simulink model "ng_pv_dynamic_dbus_p_1_sm_ng"  (Simulink 8.8)
settings: Solver=ode4  StartTime=0.0  StopTime=inf  FixedStep=0.000125  RelTol=1e-3  EnableMultiTasking=on
PreLoadFcn:
  | Ts=125e-6;Core_Num = 0; np=1; nq=1; Vmin=.9;
PostLoadFcn:
  | Ts=125e-6;Core_Num = 0; np=1; nq=1; Vmin=.9;
InitFcn:
  | Ts=125e-6;Core_Num = 0; np=1; nq=1; Vmin=.9;
undefined symbols (not defined in the file or in its folder): another_event_name, DiscIntNeverNeededParam, I, j, Left, my_event_name, Right, type, V, X
libraries: powerlib x316, simulink_extras x78, powerlib_meascontrol x47, ssn_lib x9, opal_lib x5, powerlib_extras x3, simulink x3, artemis x1, rtio_opalrt_ml605ex1 x1, rtlab x1, rtio_spectracom x1
(part 3 of 11)

== system ng_pv_dynamic_dbus_p_1_sm_ng/SM_NG/Dynamic Load BCDC1 ==
  P : Inport
  Q : Inport  Port=2
  Ground27 : powerlib/Elements/Ground  LConnTagsString=a
  Single-Phase Dynamic Load1 : Subsystem  DialogController=POWERSYS.PowerSysDialog  mask(Single-Phase Dynamic Load){NominalVoltage=|, ActiveReactivePowers=[664828.3847 359143.0862], PositiveSequence=[1 0], ExternalControl=on, NpNq=[np nq], TimeConstants=[0  0  0  0], MinimumVoltage=Vmin, LoadFlowParameters=[4,0,0,0,0]}
      mask NominalVoltage=|
      | [7967.4337
      | 60]
      mask prompts: NominalVoltage "Nominal voltage and frequency  [Vn(Vrms) fn(Hz)]:"; ActiveReactivePowers "Active and reactive power at initial voltage [Po(W) Qo(var)]:"; PositiveSequence "Initial voltage Vo [Mag(pu) Phase (deg.)]:"; ExternalControl "External control of PQ"; NpNq "Parameters [ np  nq ]:"; TimeConstants "Time constants [Tp1 Tp2 Tq1 Tq2]  (s):"; MinimumVoltage "Minimum voltage Vmin (pu):"; LoadFlowParameters "Load Flow parameters"
      mask help:
      | Implements a single-phase dynamic load. Active  power P and reactive
      | power Q absorbed by the load vary as function of voltage V  according to the
      | following equations:
      |
      |   If V>Vmin, P and Q vary as follows:
      |        P = Po * (V/Vo)^np * (1+Tp1.s)/(1+Tp2.s)
      |        Q = Qo * (V/Vo)^nq * (1+Tq1.s)/(1+Tq2.s)
      |   if V<Vmin
      |      Same equations with np=nq=2 (constant impedance load)
      mask init: same as ng_pv_dynamic_dbus_p_1_sm_ng/SM_NG/Single-Phase Dynamic Load32
      mask Help: helpview(psbhelp)
      mask Callback ExternalControl: powericon('ThreePhaseDynamicLoadCback',gcb);
      mask Display:
      | plot(-45,-45,45,45,[0,9,18,24,29,30,29,24,18,9,0,-9,-18,-24,-29,-30,-29,-24,-18,-9,0]*.9,[30,29,24,18,9,0,-9,-18,-24,-29,-30,-29,-24,-18,-9,0,9,18,24,29,30]*.9)
      | plot([0,0,10,0,-10,0]*1.1,[15,-5,-5,-15,-5,-5]*1.1)
  Single-Phase Dynamic Load2 : Subsystem  DialogController=POWERSYS.PowerSysDialog  mask(Single-Phase Dynamic Load){NominalVoltage=|, ActiveReactivePowers=[192621.3908 153291.9797], PositiveSequence=[1 0], ExternalControl=on, NpNq=[np nq], TimeConstants=[0  0  0  0], MinimumVoltage=Vmin, LoadFlowParameters=[4,0,0,0,0]}
      mask NominalVoltage=|
      | [7967.4337
      | 60]
      mask prompts: NominalVoltage "Nominal voltage and frequency  [Vn(Vrms) fn(Hz)]:"; ActiveReactivePowers "Active and reactive power at initial voltage [Po(W) Qo(var)]:"; PositiveSequence "Initial voltage Vo [Mag(pu) Phase (deg.)]:"; ExternalControl "External control of PQ"; NpNq "Parameters [ np  nq ]:"; TimeConstants "Time constants [Tp1 Tp2 Tq1 Tq2]  (s):"; MinimumVoltage "Minimum voltage Vmin (pu):"; LoadFlowParameters "Load Flow parameters"
      mask help:
      | Implements a single-phase dynamic load. Active  power P and reactive
      | power Q absorbed by the load vary as function of voltage V  according to the
      | following equations:
      |
      |   If V>Vmin, P and Q vary as follows:
      |        P = Po * (V/Vo)^np * (1+Tp1.s)/(1+Tp2.s)
      |        Q = Qo * (V/Vo)^nq * (1+Tq1.s)/(1+Tq2.s)
      |   if V<Vmin
      |      Same equations with np=nq=2 (constant impedance load)
      mask init: same as ng_pv_dynamic_dbus_p_1_sm_ng/SM_NG/Single-Phase Dynamic Load32
      mask Help: helpview(psbhelp)
      mask Callback ExternalControl: powericon('ThreePhaseDynamicLoadCback',gcb);
      mask Display:
      | plot(-45,-45,45,45,[0,9,18,24,29,30,29,24,18,9,0,-9,-18,-24,-29,-30,-29,-24,-18,-9,0]*.9,[30,29,24,18,9,0,-9,-18,-24,-29,-30,-29,-24,-18,-9,0,9,18,24,29,30]*.9)
      | plot([0,0,10,0,-10,0]*1.1,[15,-5,-5,-15,-5,-5]*1.1)
  Single-Phase Dynamic Load9 : Subsystem  DialogController=POWERSYS.PowerSysDialog  mask(Single-Phase Dynamic Load){NominalVoltage=|, ActiveReactivePowers=[324233.2017 230913.2561], PositiveSequence=[1 0], ExternalControl=on, NpNq=[np nq], TimeConstants=[0  0  0  0], MinimumVoltage=Vmin, LoadFlowParameters=[4,0,0,0,0]}
      mask NominalVoltage=|
      | [7967.4337
      | 60]
      mask prompts: NominalVoltage "Nominal voltage and frequency  [Vn(Vrms) fn(Hz)]:"; ActiveReactivePowers "Active and reactive power at initial voltage [Po(W) Qo(var)]:"; PositiveSequence "Initial voltage Vo [Mag(pu) Phase (deg.)]:"; ExternalControl "External control of PQ"; NpNq "Parameters [ np  nq ]:"; TimeConstants "Time constants [Tp1 Tp2 Tq1 Tq2]  (s):"; MinimumVoltage "Minimum voltage Vmin (pu):"; LoadFlowParameters "Load Flow parameters"
      mask help:
      | Implements a single-phase dynamic load. Active  power P and reactive
      | power Q absorbed by the load vary as function of voltage V  according to the
      | following equations:
      |
      |   If V>Vmin, P and Q vary as follows:
      |        P = Po * (V/Vo)^np * (1+Tp1.s)/(1+Tp2.s)
      |        Q = Qo * (V/Vo)^nq * (1+Tq1.s)/(1+Tq2.s)
      |   if V<Vmin
      |      Same equations with np=nq=2 (constant impedance load)
      mask init: same as ng_pv_dynamic_dbus_p_1_sm_ng/SM_NG/Single-Phase Dynamic Load32
      mask Help: helpview(psbhelp)
      mask Callback ExternalControl: powericon('ThreePhaseDynamicLoadCback',gcb);
      mask Display:
      | plot(-45,-45,45,45,[0,9,18,24,29,30,29,24,18,9,0,-9,-18,-24,-29,-30,-29,-24,-18,-9,0]*.9,[30,29,24,18,9,0,-9,-18,-24,-29,-30,-29,-24,-18,-9,0,9,18,24,29,30]*.9)
      | plot([0,0,10,0,-10,0]*1.1,[15,-5,-5,-15,-5,-5]*1.1)
  A : PMIOPort  Port=1  Side=Right
  B : PMIOPort  Port=2  Side=Right
  C : PMIOPort  Port=3  Side=Right
  wires:
  P/1 -> Single-Phase Dynamic Load2/1(P), Single-Phase Dynamic Load1/1(P), Single-Phase Dynamic Load9/1(P)
  Q/1 -> Single-Phase Dynamic Load1/2(Q), Single-Phase Dynamic Load2/2(Q), Single-Phase Dynamic Load9/2(Q)
  connections:
  Single-Phase Dynamic Load9/LConn2 -- Single-Phase Dynamic Load1/LConn2 -- Ground27/LConn1 -- Single-Phase Dynamic Load2/LConn2
  A/RConn1 -- Single-Phase Dynamic Load9/LConn1
  Single-Phase Dynamic Load2/LConn1 -- C/RConn1
  Single-Phase Dynamic Load1/LConn1 -- B/RConn1

== system ng_pv_dynamic_dbus_p_1_sm_ng/SM_NG/Dynamic Load BCDC2 ==
  P : Inport
  Q : Inport  Port=2
  Ground27 : powerlib/Elements/Ground  LConnTagsString=a
  Single-Phase Dynamic Load1 : Subsystem  DialogController=POWERSYS.PowerSysDialog  mask(Single-Phase Dynamic Load){NominalVoltage=|, ActiveReactivePowers=[934247.1199 467237.5312], PositiveSequence=[1 0], ExternalControl=on, NpNq=[np nq], TimeConstants=[0  0  0  0], MinimumVoltage=Vmin, LoadFlowParameters=[4,0,0,0,0]}
      mask NominalVoltage=|
      | [7967.4337
      | 60]
      mask prompts: NominalVoltage "Nominal voltage and frequency  [Vn(Vrms) fn(Hz)]:"; ActiveReactivePowers "Active and reactive power at initial voltage [Po(W) Qo(var)]:"; PositiveSequence "Initial voltage Vo [Mag(pu) Phase (deg.)]:"; ExternalControl "External control of PQ"; NpNq "Parameters [ np  nq ]:"; TimeConstants "Time constants [Tp1 Tp2 Tq1 Tq2]  (s):"; MinimumVoltage "Minimum voltage Vmin (pu):"; LoadFlowParameters "Load Flow parameters"
      mask help:
      | Implements a single-phase dynamic load. Active  power P and reactive
      | power Q absorbed by the load vary as function of voltage V  according to the
      | following equations:
      |
      |   If V>Vmin, P and Q vary as follows:
      |        P = Po * (V/Vo)^np * (1+Tp1.s)/(1+Tp2.s)
      |        Q = Qo * (V/Vo)^nq * (1+Tq1.s)/(1+Tq2.s)
      |   if V<Vmin
      |      Same equations with np=nq=2 (constant impedance load)
      mask init: same as ng_pv_dynamic_dbus_p_1_sm_ng/SM_NG/Single-Phase Dynamic Load32
      mask Help: helpview(psbhelp)
      mask Callback ExternalControl: powericon('ThreePhaseDynamicLoadCback',gcb);
      mask Display:
      | plot(-45,-45,45,45,[0,9,18,24,29,30,29,24,18,9,0,-9,-18,-24,-29,-30,-29,-24,-18,-9,0]*.9,[30,29,24,18,9,0,-9,-18,-24,-29,-30,-29,-24,-18,-9,0,9,18,24,29,30]*.9)
      | plot([0,0,10,0,-10,0]*1.1,[15,-5,-5,-15,-5,-5]*1.1)
  Single-Phase Dynamic Load2 : Subsystem  DialogController=POWERSYS.PowerSysDialog  mask(Single-Phase Dynamic Load){NominalVoltage=|, ActiveReactivePowers=[586764.5672 402164.5376], PositiveSequence=[1 0], ExternalControl=on, NpNq=[np nq], TimeConstants=[0  0  0  0], MinimumVoltage=Vmin, LoadFlowParameters=[4,0,0,0,0]}
      mask NominalVoltage=|
      | [7967.4337
      | 60]
      mask prompts: NominalVoltage "Nominal voltage and frequency  [Vn(Vrms) fn(Hz)]:"; ActiveReactivePowers "Active and reactive power at initial voltage [Po(W) Qo(var)]:"; PositiveSequence "Initial voltage Vo [Mag(pu) Phase (deg.)]:"; ExternalControl "External control of PQ"; NpNq "Parameters [ np  nq ]:"; TimeConstants "Time constants [Tp1 Tp2 Tq1 Tq2]  (s):"; MinimumVoltage "Minimum voltage Vmin (pu):"; LoadFlowParameters "Load Flow parameters"
      mask help:
      | Implements a single-phase dynamic load. Active  power P and reactive
      | power Q absorbed by the load vary as function of voltage V  according to the
      | following equations:
      |
      |   If V>Vmin, P and Q vary as follows:
      |        P = Po * (V/Vo)^np * (1+Tp1.s)/(1+Tp2.s)
      |        Q = Qo * (V/Vo)^nq * (1+Tq1.s)/(1+Tq2.s)
      |   if V<Vmin
      |      Same equations with np=nq=2 (constant impedance load)
      mask init: same as ng_pv_dynamic_dbus_p_1_sm_ng/SM_NG/Single-Phase Dynamic Load32
      mask Help: helpview(psbhelp)
      mask Callback ExternalControl: powericon('ThreePhaseDynamicLoadCback',gcb);
      mask Display:
      | plot(-45,-45,45,45,[0,9,18,24,29,30,29,24,18,9,0,-9,-18,-24,-29,-30,-29,-24,-18,-9,0]*.9,[30,29,24,18,9,0,-9,-18,-24,-29,-30,-29,-24,-18,-9,0,9,18,24,29,30]*.9)
      | plot([0,0,10,0,-10,0]*1.1,[15,-5,-5,-15,-5,-5]*1.1)
  Single-Phase Dynamic Load9 : Subsystem  DialogController=POWERSYS.PowerSysDialog  mask(Single-Phase Dynamic Load){NominalVoltage=|, ActiveReactivePowers=[473340.7231 336359.2548], PositiveSequence=[1 0], ExternalControl=on, NpNq=[np nq], TimeConstants=[0  0  0  0], MinimumVoltage=Vmin, LoadFlowParameters=[4,0,0,0,0]}
      mask NominalVoltage=|
      | [7967.4337
      | 60]
      mask prompts: NominalVoltage "Nominal voltage and frequency  [Vn(Vrms) fn(Hz)]:"; ActiveReactivePowers "Active and reactive power at initial voltage [Po(W) Qo(var)]:"; PositiveSequence "Initial voltage Vo [Mag(pu) Phase (deg.)]:"; ExternalControl "External control of PQ"; NpNq "Parameters [ np  nq ]:"; TimeConstants "Time constants [Tp1 Tp2 Tq1 Tq2]  (s):"; MinimumVoltage "Minimum voltage Vmin (pu):"; LoadFlowParameters "Load Flow parameters"
      mask help:
      | Implements a single-phase dynamic load. Active  power P and reactive
      | power Q absorbed by the load vary as function of voltage V  according to the
      | following equations:
      |
      |   If V>Vmin, P and Q vary as follows:
      |        P = Po * (V/Vo)^np * (1+Tp1.s)/(1+Tp2.s)
      |        Q = Qo * (V/Vo)^nq * (1+Tq1.s)/(1+Tq2.s)
      |   if V<Vmin
      |      Same equations with np=nq=2 (constant impedance load)
      mask init: same as ng_pv_dynamic_dbus_p_1_sm_ng/SM_NG/Single-Phase Dynamic Load32
      mask Help: helpview(psbhelp)
      mask Callback ExternalControl: powericon('ThreePhaseDynamicLoadCback',gcb);
      mask Display:
      | plot(-45,-45,45,45,[0,9,18,24,29,30,29,24,18,9,0,-9,-18,-24,-29,-30,-29,-24,-18,-9,0]*.9,[30,29,24,18,9,0,-9,-18,-24,-29,-30,-29,-24,-18,-9,0,9,18,24,29,30]*.9)
      | plot([0,0,10,0,-10,0]*1.1,[15,-5,-5,-15,-5,-5]*1.1)
  A : PMIOPort  Port=1  Side=Right
  B : PMIOPort  Port=2  Side=Right
  C : PMIOPort  Port=3  Side=Right
  wires:
  P/1 -> Single-Phase Dynamic Load2/1(P), Single-Phase Dynamic Load1/1(P), Single-Phase Dynamic Load9/1(P)
  Q/1 -> Single-Phase Dynamic Load1/2(Q), Single-Phase Dynamic Load2/2(Q), Single-Phase Dynamic Load9/2(Q)
  connections:
  Single-Phase Dynamic Load9/LConn2 -- Single-Phase Dynamic Load1/LConn2 -- Ground27/LConn1 -- Single-Phase Dynamic Load2/LConn2
  A/RConn1 -- Single-Phase Dynamic Load9/LConn1
  Single-Phase Dynamic Load2/LConn1 -- C/RConn1
  Single-Phase Dynamic Load1/LConn1 -- B/RConn1

== system ng_pv_dynamic_dbus_p_1_sm_ng/SM_NG/Dynamic Load BCDC3 ==
  P : Inport
  Q : Inport  Port=2
  Ground27 : powerlib/Elements/Ground  LConnTagsString=a
  Single-Phase Dynamic Load1 : Subsystem  DialogController=POWERSYS.PowerSysDialog  mask(Single-Phase Dynamic Load){NominalVoltage=|, ActiveReactivePowers=[359272.8363 164258.4315], PositiveSequence=[1 0], ExternalControl=on, NpNq=[np nq], TimeConstants=[0  0  0  0], MinimumVoltage=Vmin, LoadFlowParameters=[4,0,0,0,0]}
      mask NominalVoltage=|
      | [7967.4337
      | 60]
      mask prompts: NominalVoltage "Nominal voltage and frequency  [Vn(Vrms) fn(Hz)]:"; ActiveReactivePowers "Active and reactive power at initial voltage [Po(W) Qo(var)]:"; PositiveSequence "Initial voltage Vo [Mag(pu) Phase (deg.)]:"; ExternalControl "External control of PQ"; NpNq "Parameters [ np  nq ]:"; TimeConstants "Time constants [Tp1 Tp2 Tq1 Tq2]  (s):"; MinimumVoltage "Minimum voltage Vmin (pu):"; LoadFlowParameters "Load Flow parameters"
      mask help:
      | Implements a single-phase dynamic load. Active  power P and reactive
      | power Q absorbed by the load vary as function of voltage V  according to the
      | following equations:
      |
      |   If V>Vmin, P and Q vary as follows:
      |        P = Po * (V/Vo)^np * (1+Tp1.s)/(1+Tp2.s)
      |        Q = Qo * (V/Vo)^nq * (1+Tq1.s)/(1+Tq2.s)
      |   if V<Vmin
      |      Same equations with np=nq=2 (constant impedance load)
      mask init: same as ng_pv_dynamic_dbus_p_1_sm_ng/SM_NG/Single-Phase Dynamic Load32
      mask Help: helpview(psbhelp)
      mask Callback ExternalControl: powericon('ThreePhaseDynamicLoadCback',gcb);
      mask Display:
      | plot(-45,-45,45,45,[0,9,18,24,29,30,29,24,18,9,0,-9,-18,-24,-29,-30,-29,-24,-18,-9,0]*.9,[30,29,24,18,9,0,-9,-18,-24,-29,-30,-29,-24,-18,-9,0,9,18,24,29,30]*.9)
      | plot([0,0,10,0,-10,0]*1.1,[15,-5,-5,-15,-5,-5]*1.1)
  Single-Phase Dynamic Load2 : Subsystem  DialogController=POWERSYS.PowerSysDialog  mask(Single-Phase Dynamic Load){NominalVoltage=|, ActiveReactivePowers=[167826.2591 104736.8385], PositiveSequence=[1 0], ExternalControl=on, NpNq=[np nq], TimeConstants=[0  0  0  0], MinimumVoltage=Vmin, LoadFlowParameters=[4,0,0,0,0]}
      mask NominalVoltage=|
      | [7967.4337
      | 60]
      mask prompts: NominalVoltage "Nominal voltage and frequency  [Vn(Vrms) fn(Hz)]:"; ActiveReactivePowers "Active and reactive power at initial voltage [Po(W) Qo(var)]:"; PositiveSequence "Initial voltage Vo [Mag(pu) Phase (deg.)]:"; ExternalControl "External control of PQ"; NpNq "Parameters [ np  nq ]:"; TimeConstants "Time constants [Tp1 Tp2 Tq1 Tq2]  (s):"; MinimumVoltage "Minimum voltage Vmin (pu):"; LoadFlowParameters "Load Flow parameters"
      mask help:
      | Implements a single-phase dynamic load. Active  power P and reactive
      | power Q absorbed by the load vary as function of voltage V  according to the
      | following equations:
      |
      |   If V>Vmin, P and Q vary as follows:
      |        P = Po * (V/Vo)^np * (1+Tp1.s)/(1+Tp2.s)
      |        Q = Qo * (V/Vo)^nq * (1+Tq1.s)/(1+Tq2.s)
      |   if V<Vmin
      |      Same equations with np=nq=2 (constant impedance load)
      mask init: same as ng_pv_dynamic_dbus_p_1_sm_ng/SM_NG/Single-Phase Dynamic Load32
      mask Help: helpview(psbhelp)
      mask Callback ExternalControl: powericon('ThreePhaseDynamicLoadCback',gcb);
      mask Display:
      | plot(-45,-45,45,45,[0,9,18,24,29,30,29,24,18,9,0,-9,-18,-24,-29,-30,-29,-24,-18,-9,0]*.9,[30,29,24,18,9,0,-9,-18,-24,-29,-30,-29,-24,-18,-9,0,9,18,24,29,30]*.9)
      | plot([0,0,10,0,-10,0]*1.1,[15,-5,-5,-15,-5,-5]*1.1)
  Single-Phase Dynamic Load9 : Subsystem  DialogController=POWERSYS.PowerSysDialog  mask(Single-Phase Dynamic Load){NominalVoltage=|, ActiveReactivePowers=[330455.6138 202114.2565], PositiveSequence=[1 0], ExternalControl=on, NpNq=[np nq], TimeConstants=[0  0  0  0], MinimumVoltage=Vmin, LoadFlowParameters=[4,0,0,0,0]}
      mask NominalVoltage=|
      | [7967.4337
      | 60]
      mask prompts: NominalVoltage "Nominal voltage and frequency  [Vn(Vrms) fn(Hz)]:"; ActiveReactivePowers "Active and reactive power at initial voltage [Po(W) Qo(var)]:"; PositiveSequence "Initial voltage Vo [Mag(pu) Phase (deg.)]:"; ExternalControl "External control of PQ"; NpNq "Parameters [ np  nq ]:"; TimeConstants "Time constants [Tp1 Tp2 Tq1 Tq2]  (s):"; MinimumVoltage "Minimum voltage Vmin (pu):"; LoadFlowParameters "Load Flow parameters"
      mask help:
      | Implements a single-phase dynamic load. Active  power P and reactive
      | power Q absorbed by the load vary as function of voltage V  according to the
      | following equations:
      |
      |   If V>Vmin, P and Q vary as follows:
      |        P = Po * (V/Vo)^np * (1+Tp1.s)/(1+Tp2.s)
      |        Q = Qo * (V/Vo)^nq * (1+Tq1.s)/(1+Tq2.s)
      |   if V<Vmin
      |      Same equations with np=nq=2 (constant impedance load)
      mask init: same as ng_pv_dynamic_dbus_p_1_sm_ng/SM_NG/Single-Phase Dynamic Load32
      mask Help: helpview(psbhelp)
      mask Callback ExternalControl: powericon('ThreePhaseDynamicLoadCback',gcb);
      mask Display:
      | plot(-45,-45,45,45,[0,9,18,24,29,30,29,24,18,9,0,-9,-18,-24,-29,-30,-29,-24,-18,-9,0]*.9,[30,29,24,18,9,0,-9,-18,-24,-29,-30,-29,-24,-18,-9,0,9,18,24,29,30]*.9)
      | plot([0,0,10,0,-10,0]*1.1,[15,-5,-5,-15,-5,-5]*1.1)
  A : PMIOPort  Port=1  Side=Right
  B : PMIOPort  Port=2  Side=Right
  C : PMIOPort  Port=3  Side=Right
  wires:
  P/1 -> Single-Phase Dynamic Load2/1(P), Single-Phase Dynamic Load1/1(P), Single-Phase Dynamic Load9/1(P)
  Q/1 -> Single-Phase Dynamic Load1/2(Q), Single-Phase Dynamic Load2/2(Q), Single-Phase Dynamic Load9/2(Q)
  connections:
  Single-Phase Dynamic Load9/LConn2 -- Single-Phase Dynamic Load1/LConn2 -- Ground27/LConn1 -- Single-Phase Dynamic Load2/LConn2
  A/RConn1 -- Single-Phase Dynamic Load9/LConn1
  Single-Phase Dynamic Load2/LConn1 -- C/RConn1
  Single-Phase Dynamic Load1/LConn1 -- B/RConn1

== system ng_pv_dynamic_dbus_p_1_sm_ng/SM_NG/IED10 ==
  Current Measurement : powerlib/Measurements/Current Measurement  PhasorSimulation=off  OutputType=Complex  PSBequivalent=0
  Ground1 : powerlib/Elements/Ground  LConnTagsString=a
  Voltage Measurement : powerlib/Measurements/Voltage Measurement  PhasorSimulation=off  OutputType=Complex  PSBequivalent=0
  A : PMIOPort  Port=1  Side=Right
  a : PMIOPort  Port=2  Side=Left
  tag scope: I_IED10=global, V_IED10=global
  wires:
  Current Measurement/1 -> [I_IED10]
  Voltage Measurement/1 -> [V_IED10]
  connections:
  Ground1/LConn1 -- Voltage Measurement/LConn2
  Current Measurement/LConn1 -- a/RConn1
  Voltage Measurement/LConn1 -- A/RConn1 -- Current Measurement/RConn1

== system ng_pv_dynamic_dbus_p_1_sm_ng/SM_NG/IED14A ==
  Current Measurement : powerlib/Measurements/Current Measurement  PhasorSimulation=off  OutputType=Complex  PSBequivalent=0
  Ground1 : powerlib/Elements/Ground  LConnTagsString=a
  Voltage Measurement : powerlib/Measurements/Voltage Measurement  PhasorSimulation=off  OutputType=Complex  PSBequivalent=0
  A : PMIOPort  Port=1  Side=Right
  a : PMIOPort  Port=2  Side=Left
  tag scope: I_IED14A=global, V_IED14A=global
  wires:
  Current Measurement/1 -> [I_IED14A]
  Voltage Measurement/1 -> [V_IED14A]
  connections:
  Ground1/LConn1 -- Voltage Measurement/LConn2
  Current Measurement/LConn1 -- a/RConn1
  Voltage Measurement/LConn1 -- A/RConn1 -- Current Measurement/RConn1

== system ng_pv_dynamic_dbus_p_1_sm_ng/SM_NG/IED7A ==
  Current Measurement : powerlib/Measurements/Current Measurement  PhasorSimulation=off  OutputType=Complex  PSBequivalent=0
  Ground1 : powerlib/Elements/Ground  LConnTagsString=a
  Voltage Measurement : powerlib/Measurements/Voltage Measurement  PhasorSimulation=off  OutputType=Complex  PSBequivalent=0
  A : PMIOPort  Port=1  Side=Right
  a : PMIOPort  Port=2  Side=Left
  tag scope: I_IED7A=global, V_IED7A=global
  wires:
  Current Measurement/1 -> [I_IED7A]
  Voltage Measurement/1 -> [V_IED7A]
  connections:
  Ground1/LConn1 -- Voltage Measurement/LConn2
  Current Measurement/LConn1 -- a/RConn1
  Voltage Measurement/LConn1 -- A/RConn1 -- Current Measurement/RConn1

== system ng_pv_dynamic_dbus_p_1_sm_ng/SM_NG/PV11 ==
  PQ : Inport
  -Q : Gain  Gain=-1  SaturateOnIntegerOverflow=on  OutDataTypeStr=Inherit: Same as input  ParamDataTypeStr=Inherit: Same as input
  Dynamic Load : powerlib/Elements/Three-Phase Dynamic Load  NominalVoltage=[13800.00 60 ]  ActiveReactivePowers=|  PositiveSequence=[0.994 -11.8]  ExternalControl=on  NpNq=[np nq]  TimeConstants="[0  0  0  0]"  MinimumVoltage=Vmin  Tfilter=1e-4  LoadFlowParameters=[4,0,0,0,0]
      | [-684000.00
      | 0]
  a : PMIOPort  Port=1  Side=Right
  b : PMIOPort  Port=2  Side=Right
  c : PMIOPort  Port=3  Side=Right
  wires:
  PQ/1 -> -Q/1
  -Q/1 -> Dynamic Load/1
  connections:
  a/RConn1 -- Dynamic Load/LConn1
  c/RConn1 -- Dynamic Load/LConn3
  b/RConn1 -- Dynamic Load/LConn2

== system ng_pv_dynamic_dbus_p_1_sm_ng/SM_NG/Single-Phase Dynamic Load30 ==
  PQ : Inport
  Controlled Current Source : powerlib/Electrical Sources/Controlled Current Source  Initialize=on  Source_Type=AC  Amplitude=0  Phase=0  Frequency=0  Measurements=None
  Ground50 : powerlib/Elements/Ground  LConnTagsString=a
  Voltage Measurement1 : powerlib/Measurements/Voltage Measurement  PhasorSimulation=off  OutputType=Complex  PSBequivalent=0
  model : Subsystem
  a : PMIOPort  Tag=PMCPort  Port=1  Side=Right
  wires:
  PQ/1 -> model/2(PQ)
  Voltage Measurement1/1 -> model/1(v)
  model/1(i) -> Controlled Current Source/1
  connections:
  Controlled Current Source/RConn1 -- Voltage Measurement1/LConn1 -- a/RConn1
  Controlled Current Source/LConn1 -- Ground50/LConn1 -- Voltage Measurement1/LConn2

== system ng_pv_dynamic_dbus_p_1_sm_ng/SM_NG/Single-Phase Dynamic Load32 ==
  PQ : Inport
  Controlled Current Source : powerlib/Electrical Sources/Controlled Current Source  Initialize=on  Source_Type=AC  Amplitude=0  Phase=0  Frequency=0  Measurements=None
  Ground52 : powerlib/Elements/Ground  LConnTagsString=a
  Voltage Measurement1 : powerlib/Measurements/Voltage Measurement  PhasorSimulation=off  OutputType=Complex  PSBequivalent=0
  model : Subsystem
  a : PMIOPort  Tag=PMCPort  Port=1  Side=Right
  wires:
  PQ/1 -> model/2(PQ)
  Voltage Measurement1/1 -> model/1(v)
  model/1(i) -> Controlled Current Source/1
  connections:
  Voltage Measurement1/LConn1 -- a/RConn1 -- Controlled Current Source/RConn1
  Voltage Measurement1/LConn2 -- Controlled Current Source/LConn1 -- Ground52/LConn1

== system ng_pv_dynamic_dbus_p_1_sm_ng/SM_NG/Single-Phase Dynamic Load33 ==
  PQ : Inport
  Controlled Current Source : powerlib/Electrical Sources/Controlled Current Source  Initialize=on  Source_Type=AC  Amplitude=0  Phase=0  Frequency=0  Measurements=None
  Ground52 : powerlib/Elements/Ground  LConnTagsString=a
  Voltage Measurement1 : powerlib/Measurements/Voltage Measurement  PhasorSimulation=off  OutputType=Complex  PSBequivalent=0
  model : Subsystem
  a : PMIOPort  Tag=PMCPort  Port=1  Side=Right
  wires:
  PQ/1 -> model/2(PQ)
  Voltage Measurement1/1 -> model/1(v)
  model/1(i) -> Controlled Current Source/1
  connections:
  Voltage Measurement1/LConn1 -- a/RConn1 -- Controlled Current Source/RConn1
  Voltage Measurement1/LConn2 -- Ground52/LConn1 -- Controlled Current Source/LConn1

== system ng_pv_dynamic_dbus_p_1_sm_ng/SM_NG/Single-Phase Dynamic Load34 ==
  PQ : Inport
  Controlled Current Source : powerlib/Electrical Sources/Controlled Current Source  Initialize=on  Source_Type=AC  Amplitude=0  Phase=0  Frequency=0  Measurements=None
  Ground52 : powerlib/Elements/Ground  LConnTagsString=a
  Voltage Measurement1 : powerlib/Measurements/Voltage Measurement  PhasorSimulation=off  OutputType=Complex  PSBequivalent=0
  model : Subsystem
  a : PMIOPort  Tag=PMCPort  Port=1  Side=Right
  wires:
  PQ/1 -> model/2(PQ)
  Voltage Measurement1/1 -> model/1(v)
  model/1(i) -> Controlled Current Source/1
  connections:
  Voltage Measurement1/LConn1 -- a/RConn1 -- Controlled Current Source/RConn1
  Voltage Measurement1/LConn2 -- Ground52/LConn1 -- Controlled Current Source/LConn1

== system ng_pv_dynamic_dbus_p_1_sm_ng/SM_NG/Single-Phase Dynamic Load35 ==
  PQ : Inport
  Controlled Current Source : powerlib/Electrical Sources/Controlled Current Source  Initialize=on  Source_Type=AC  Amplitude=0  Phase=0  Frequency=0  Measurements=None
  Ground52 : powerlib/Elements/Ground  LConnTagsString=a
  Voltage Measurement1 : powerlib/Measurements/Voltage Measurement  PhasorSimulation=off  OutputType=Complex  PSBequivalent=0
  model : Subsystem
  a : PMIOPort  Tag=PMCPort  Port=1  Side=Right
  wires:
  PQ/1 -> model/2(PQ)
  Voltage Measurement1/1 -> model/1(v)
  model/1(i) -> Controlled Current Source/1
  connections:
  Voltage Measurement1/LConn1 -- a/RConn1 -- Controlled Current Source/RConn1
  Voltage Measurement1/LConn2 -- Controlled Current Source/LConn1 -- Ground52/LConn1

== system ng_pv_dynamic_dbus_p_1_sm_ng/SM_NG/Single-Phase Dynamic Load36 ==
  PQ : Inport
  Controlled Current Source : powerlib/Electrical Sources/Controlled Current Source  Initialize=on  Source_Type=AC  Amplitude=0  Phase=0  Frequency=0  Measurements=None
  Ground52 : powerlib/Elements/Ground  LConnTagsString=a
  Voltage Measurement1 : powerlib/Measurements/Voltage Measurement  PhasorSimulation=off  OutputType=Complex  PSBequivalent=0
  model : Subsystem
  a : PMIOPort  Tag=PMCPort  Port=1  Side=Right
  wires:
  PQ/1 -> model/2(PQ)
  Voltage Measurement1/1 -> model/1(v)
  model/1(i) -> Controlled Current Source/1
  connections:
  Voltage Measurement1/LConn1 -- a/RConn1 -- Controlled Current Source/RConn1
  Voltage Measurement1/LConn2 -- Ground52/LConn1 -- Controlled Current Source/LConn1

== system ng_pv_dynamic_dbus_p_1_sm_ng/SM_NG/Single-Phase Dynamic Load37 ==
  PQ : Inport
  Controlled Current Source : powerlib/Electrical Sources/Controlled Current Source  Initialize=on  Source_Type=AC  Amplitude=0  Phase=0  Frequency=0  Measurements=None
  Ground52 : powerlib/Elements/Ground  LConnTagsString=a
  Voltage Measurement1 : powerlib/Measurements/Voltage Measurement  PhasorSimulation=off  OutputType=Complex  PSBequivalent=0
  model : Subsystem
  a : PMIOPort  Tag=PMCPort  Port=1  Side=Right
  wires:
  PQ/1 -> model/2(PQ)
  Voltage Measurement1/1 -> model/1(v)
  model/1(i) -> Controlled Current Source/1
  connections:
  Voltage Measurement1/LConn1 -- a/RConn1 -- Controlled Current Source/RConn1
  Ground52/LConn1 -- Voltage Measurement1/LConn2 -- Controlled Current Source/LConn1

== system ng_pv_dynamic_dbus_p_1_sm_ng/SM_NG/Single-Phase Dynamic Load38 ==
  PQ : Inport
  Controlled Current Source : powerlib/Electrical Sources/Controlled Current Source  Initialize=on  Source_Type=AC  Amplitude=0  Phase=0  Frequency=0  Measurements=None
  Ground52 : powerlib/Elements/Ground  LConnTagsString=a
  Voltage Measurement1 : powerlib/Measurements/Voltage Measurement  PhasorSimulation=off  OutputType=Complex  PSBequivalent=0
  model : Subsystem
  a : PMIOPort  Tag=PMCPort  Port=1  Side=Right
  wires:
  PQ/1 -> model/2(PQ)
  Voltage Measurement1/1 -> model/1(v)
  model/1(i) -> Controlled Current Source/1
  connections:
  Voltage Measurement1/LConn1 -- a/RConn1 -- Controlled Current Source/RConn1
  Voltage Measurement1/LConn2 -- Ground52/LConn1 -- Controlled Current Source/LConn1

== system ng_pv_dynamic_dbus_p_1_sm_ng/SM_NG/Single-Phase Dynamic Load39 ==
  PQ : Inport
  Controlled Current Source : powerlib/Electrical Sources/Controlled Current Source  Initialize=on  Source_Type=AC  Amplitude=0  Phase=0  Frequency=0  Measurements=None
  Ground52 : powerlib/Elements/Ground  LConnTagsString=a
  Voltage Measurement1 : powerlib/Measurements/Voltage Measurement  PhasorSimulation=off  OutputType=Complex  PSBequivalent=0
  model : Subsystem
  a : PMIOPort  Tag=PMCPort  Port=1  Side=Right
  wires:
  PQ/1 -> model/2(PQ)
  Voltage Measurement1/1 -> model/1(v)
  model/1(i) -> Controlled Current Source/1
  connections:
  Voltage Measurement1/LConn1 -- a/RConn1 -- Controlled Current Source/RConn1
  Voltage Measurement1/LConn2 -- Ground52/LConn1 -- Controlled Current Source/LConn1

== system ng_pv_dynamic_dbus_p_1_sm_ng/SM_NG/Single-Phase Dynamic Load40 ==
  PQ : Inport
  Controlled Current Source : powerlib/Electrical Sources/Controlled Current Source  Initialize=on  Source_Type=AC  Amplitude=0  Phase=0  Frequency=0  Measurements=None
  Ground57 : powerlib/Elements/Ground  LConnTagsString=a
  Voltage Measurement1 : powerlib/Measurements/Voltage Measurement  PhasorSimulation=off  OutputType=Complex  PSBequivalent=0
  model : Subsystem
  a : PMIOPort  Tag=PMCPort  Port=1  Side=Right
  wires:
  PQ/1 -> model/2(PQ)
  Voltage Measurement1/1 -> model/1(v)
  model/1(i) -> Controlled Current Source/1
  connections:
  Voltage Measurement1/LConn1 -- a/RConn1 -- Controlled Current Source/RConn1
  Voltage Measurement1/LConn2 -- Ground57/LConn1 -- Controlled Current Source/LConn1

== system ng_pv_dynamic_dbus_p_1_sm_ng/SM_NG/Single-Phase Dynamic Load41 ==
  PQ : Inport
  Controlled Current Source : powerlib/Electrical Sources/Controlled Current Source  Initialize=on  Source_Type=AC  Amplitude=0  Phase=0  Frequency=0  Measurements=None
  Ground57 : powerlib/Elements/Ground  LConnTagsString=a
  Voltage Measurement1 : powerlib/Measurements/Voltage Measurement  PhasorSimulation=off  OutputType=Complex  PSBequivalent=0
  model : Subsystem
  a : PMIOPort  Tag=PMCPort  Port=1  Side=Right
  wires:
  PQ/1 -> model/2(PQ)
  Voltage Measurement1/1 -> model/1(v)
  model/1(i) -> Controlled Current Source/1
  connections:
  Voltage Measurement1/LConn1 -- a/RConn1 -- Controlled Current Source/RConn1
  Voltage Measurement1/LConn2 -- Ground57/LConn1 -- Controlled Current Source/LConn1

== system ng_pv_dynamic_dbus_p_1_sm_ng/SM_NG/Single-Phase Dynamic Load42 ==
  PQ : Inport
  Controlled Current Source : powerlib/Electrical Sources/Controlled Current Source  Initialize=on  Source_Type=AC  Amplitude=0  Phase=0  Frequency=0  Measurements=None
  Ground50 : powerlib/Elements/Ground  LConnTagsString=a
  Voltage Measurement1 : powerlib/Measurements/Voltage Measurement  PhasorSimulation=off  OutputType=Complex  PSBequivalent=0
  model : Subsystem
  a : PMIOPort  Tag=PMCPort  Port=1  Side=Right
  wires:
  PQ/1 -> model/2(PQ)
  Voltage Measurement1/1 -> model/1(v)
  model/1(i) -> Controlled Current Source/1
  connections:
  Voltage Measurement1/LConn1 -- a/RConn1 -- Controlled Current Source/RConn1
  Voltage Measurement1/LConn2 -- Ground50/LConn1 -- Controlled Current Source/LConn1

== system ng_pv_dynamic_dbus_p_1_sm_ng/SM_NG/Single-Phase Dynamic Load43 ==
  PQ : Inport
  Controlled Current Source : powerlib/Electrical Sources/Controlled Current Source  Initialize=on  Source_Type=AC  Amplitude=0  Phase=0  Frequency=0  Measurements=None
  Ground57 : powerlib/Elements/Ground  LConnTagsString=a
  Voltage Measurement1 : powerlib/Measurements/Voltage Measurement  PhasorSimulation=off  OutputType=Complex  PSBequivalent=0
  model : Subsystem
  a : PMIOPort  Tag=PMCPort  Port=1  Side=Right
  wires:
  PQ/1 -> model/2(PQ)
  Voltage Measurement1/1 -> model/1(v)
  model/1(i) -> Controlled Current Source/1
  connections:
  Voltage Measurement1/LConn1 -- a/RConn1 -- Controlled Current Source/RConn1
  Voltage Measurement1/LConn2 -- Ground57/LConn1 -- Controlled Current Source/LConn1

== system ng_pv_dynamic_dbus_p_1_sm_ng/SM_NG/Single-Phase Dynamic Load44 ==
  PQ : Inport
  Controlled Current Source : powerlib/Electrical Sources/Controlled Current Source  Initialize=on  Source_Type=AC  Amplitude=0  Phase=0  Frequency=0  Measurements=None
  Ground57 : powerlib/Elements/Ground  LConnTagsString=a
  Voltage Measurement1 : powerlib/Measurements/Voltage Measurement  PhasorSimulation=off  OutputType=Complex  PSBequivalent=0
  model : Subsystem
  a : PMIOPort  Tag=PMCPort  Port=1  Side=Right
  wires:
  PQ/1 -> model/2(PQ)
  Voltage Measurement1/1 -> model/1(v)
  model/1(i) -> Controlled Current Source/1
  connections:
  Voltage Measurement1/LConn1 -- a/RConn1 -- Controlled Current Source/RConn1
  Voltage Measurement1/LConn2 -- Ground57/LConn1 -- Controlled Current Source/LConn1

== system ng_pv_dynamic_dbus_p_1_sm_ng/SM_NG/Single-Phase Dynamic Load45 ==
  PQ : Inport
  Controlled Current Source : powerlib/Electrical Sources/Controlled Current Source  Initialize=on  Source_Type=AC  Amplitude=0  Phase=0  Frequency=0  Measurements=None
  Ground57 : powerlib/Elements/Ground  LConnTagsString=a
  Voltage Measurement1 : powerlib/Measurements/Voltage Measurement  PhasorSimulation=off  OutputType=Complex  PSBequivalent=0
  model : Subsystem
  a : PMIOPort  Tag=PMCPort  Port=1  Side=Right
  wires:
  PQ/1 -> model/2(PQ)
  Voltage Measurement1/1 -> model/1(v)
  model/1(i) -> Controlled Current Source/1
  connections:
  Voltage Measurement1/LConn1 -- a/RConn1 -- Controlled Current Source/RConn1
  Voltage Measurement1/LConn2 -- Ground57/LConn1 -- Controlled Current Source/LConn1

== system ng_pv_dynamic_dbus_p_1_sm_ng/SM_NG/Single-Phase Dynamic Load46 ==
  PQ : Inport
  Controlled Current Source : powerlib/Electrical Sources/Controlled Current Source  Initialize=on  Source_Type=AC  Amplitude=0  Phase=0  Frequency=0  Measurements=None
  Ground57 : powerlib/Elements/Ground  LConnTagsString=a
  Voltage Measurement1 : powerlib/Measurements/Voltage Measurement  PhasorSimulation=off  OutputType=Complex  PSBequivalent=0
  model : Subsystem
  a : PMIOPort  Tag=PMCPort  Port=1  Side=Right
  wires:
  PQ/1 -> model/2(PQ)
  Voltage Measurement1/1 -> model/1(v)
  model/1(i) -> Controlled Current Source/1
  connections:
  Voltage Measurement1/LConn1 -- a/RConn1 -- Controlled Current Source/RConn1
  Voltage Measurement1/LConn2 -- Ground57/LConn1 -- Controlled Current Source/LConn1

== system ng_pv_dynamic_dbus_p_1_sm_ng/SM_NG/Single-Phase Dynamic Load47 ==
  PQ : Inport
  Controlled Current Source : powerlib/Electrical Sources/Controlled Current Source  Initialize=on  Source_Type=AC  Amplitude=0  Phase=0  Frequency=0  Measurements=None
  Ground52 : powerlib/Elements/Ground  LConnTagsString=a
  Voltage Measurement1 : powerlib/Measurements/Voltage Measurement  PhasorSimulation=off  OutputType=Complex  PSBequivalent=0
  model : Subsystem
  a : PMIOPort  Tag=PMCPort  Port=1  Side=Right
  wires:
  PQ/1 -> model/2(PQ)
  Voltage Measurement1/1 -> model/1(v)
  model/1(i) -> Controlled Current Source/1
  connections:
  Voltage Measurement1/LConn1 -- a/RConn1 -- Controlled Current Source/RConn1
  Voltage Measurement1/LConn2 -- Ground52/LConn1 -- Controlled Current Source/LConn1

== system ng_pv_dynamic_dbus_p_1_sm_ng/SM_NG/Single-Phase Dynamic Load48 ==
  PQ : Inport
  Controlled Current Source : powerlib/Electrical Sources/Controlled Current Source  Initialize=on  Source_Type=AC  Amplitude=0  Phase=0  Frequency=0  Measurements=None
  Ground52 : powerlib/Elements/Ground  LConnTagsString=a
  Voltage Measurement1 : powerlib/Measurements/Voltage Measurement  PhasorSimulation=off  OutputType=Complex  PSBequivalent=0
  model : Subsystem
  a : PMIOPort  Tag=PMCPort  Port=1  Side=Right
  wires:
  PQ/1 -> model/2(PQ)
  Voltage Measurement1/1 -> model/1(v)
  model/1(i) -> Controlled Current Source/1
  connections:
  Voltage Measurement1/LConn1 -- a/RConn1 -- Controlled Current Source/RConn1
  Voltage Measurement1/LConn2 -- Ground52/LConn1 -- Controlled Current Source/LConn1

== system ng_pv_dynamic_dbus_p_1_sm_ng/SM_NG/Single-Phase Dynamic Load49 ==
  PQ : Inport
  Controlled Current Source : powerlib/Electrical Sources/Controlled Current Source  Initialize=on  Source_Type=AC  Amplitude=0  Phase=0  Frequency=0  Measurements=None
  Ground52 : powerlib/Elements/Ground  LConnTagsString=a
  Voltage Measurement1 : powerlib/Measurements/Voltage Measurement  PhasorSimulation=off  OutputType=Complex  PSBequivalent=0
  model : Subsystem
  a : PMIOPort  Tag=PMCPort  Port=1  Side=Right
  wires:
  PQ/1 -> model/2(PQ)
  Voltage Measurement1/1 -> model/1(v)
  model/1(i) -> Controlled Current Source/1
  connections:
  Voltage Measurement1/LConn1 -- a/RConn1 -- Controlled Current Source/RConn1
  Voltage Measurement1/LConn2 -- Ground52/LConn1 -- Controlled Current Source/LConn1

== system ng_pv_dynamic_dbus_p_1_sm_ng/SM_NG/Single-Phase Dynamic Load50 ==
  PQ : Inport
  Controlled Current Source : powerlib/Electrical Sources/Controlled Current Source  Initialize=on  Source_Type=AC  Amplitude=0  Phase=0  Frequency=0  Measurements=None
  Ground59 : powerlib/Elements/Ground  LConnTagsString=a
  Voltage Measurement1 : powerlib/Measurements/Voltage Measurement  PhasorSimulation=off  OutputType=Complex  PSBequivalent=0
  model : Subsystem
  a : PMIOPort  Tag=PMCPort  Port=1  Side=Right
  wires:
  PQ/1 -> model/2(PQ)
  Voltage Measurement1/1 -> model/1(v)
  model/1(i) -> Controlled Current Source/1
  connections:
  Voltage Measurement1/LConn1 -- a/RConn1 -- Controlled Current Source/RConn1
  Voltage Measurement1/LConn2 -- Ground59/LConn1 -- Controlled Current Source/LConn1

== system ng_pv_dynamic_dbus_p_1_sm_ng/SM_NG/Single-Phase Dynamic Load51 ==
  PQ : Inport
  Controlled Current Source : powerlib/Electrical Sources/Controlled Current Source  Initialize=on  Source_Type=AC  Amplitude=0  Phase=0  Frequency=0  Measurements=None
  Ground59 : powerlib/Elements/Ground  LConnTagsString=a
  Voltage Measurement1 : powerlib/Measurements/Voltage Measurement  PhasorSimulation=off  OutputType=Complex  PSBequivalent=0
  model : Subsystem
  a : PMIOPort  Tag=PMCPort  Port=1  Side=Right
  wires:
  PQ/1 -> model/2(PQ)
  Voltage Measurement1/1 -> model/1(v)
  model/1(i) -> Controlled Current Source/1
  connections:
  Voltage Measurement1/LConn1 -- a/RConn1 -- Controlled Current Source/RConn1
  Voltage Measurement1/LConn2 -- Ground59/LConn1 -- Controlled Current Source/LConn1

== system ng_pv_dynamic_dbus_p_1_sm_ng/SM_NG/Single-Phase Dynamic Load52 ==
  PQ : Inport
  Controlled Current Source : powerlib/Electrical Sources/Controlled Current Source  Initialize=on  Source_Type=AC  Amplitude=0  Phase=0  Frequency=0  Measurements=None
  Ground59 : powerlib/Elements/Ground  LConnTagsString=a
  Voltage Measurement1 : powerlib/Measurements/Voltage Measurement  PhasorSimulation=off  OutputType=Complex  PSBequivalent=0
  model : Subsystem
  a : PMIOPort  Tag=PMCPort  Port=1  Side=Right
  wires:
  PQ/1 -> model/2(PQ)
  Voltage Measurement1/1 -> model/1(v)
  model/1(i) -> Controlled Current Source/1
  connections:
  Voltage Measurement1/LConn1 -- a/RConn1 -- Controlled Current Source/RConn1
  Voltage Measurement1/LConn2 -- Controlled Current Source/LConn1 -- Ground59/LConn1

== system ng_pv_dynamic_dbus_p_1_sm_ng/SM_NG/Single-Phase Dynamic Load53 ==
  PQ : Inport
  Controlled Current Source : powerlib/Electrical Sources/Controlled Current Source  Initialize=on  Source_Type=AC  Amplitude=0  Phase=0  Frequency=0  Measurements=None
  Ground62 : powerlib/Elements/Ground  LConnTagsString=a
  Voltage Measurement1 : powerlib/Measurements/Voltage Measurement  PhasorSimulation=off  OutputType=Complex  PSBequivalent=0
  model : Subsystem
  a : PMIOPort  Tag=PMCPort  Port=1  Side=Right
  wires:
  PQ/1 -> model/2(PQ)
  Voltage Measurement1/1 -> model/1(v)
  model/1(i) -> Controlled Current Source/1
  connections:
  Voltage Measurement1/LConn1 -- a/RConn1 -- Controlled Current Source/RConn1
  Voltage Measurement1/LConn2 -- Ground62/LConn1 -- Controlled Current Source/LConn1

== system ng_pv_dynamic_dbus_p_1_sm_ng/SM_NG/Single-Phase Dynamic Load54 ==
  PQ : Inport
  Controlled Current Source : powerlib/Electrical Sources/Controlled Current Source  Initialize=on  Source_Type=AC  Amplitude=0  Phase=0  Frequency=0  Measurements=None
  Ground64 : powerlib/Elements/Ground  LConnTagsString=a
  Voltage Measurement1 : powerlib/Measurements/Voltage Measurement  PhasorSimulation=off  OutputType=Complex  PSBequivalent=0
  model : Subsystem
  a : PMIOPort  Tag=PMCPort  Port=1  Side=Right
  wires:
  PQ/1 -> model/2(PQ)
  Voltage Measurement1/1 -> model/1(v)
  model/1(i) -> Controlled Current Source/1
  connections:
  Voltage Measurement1/LConn1 -- a/RConn1 -- Controlled Current Source/RConn1
  Voltage Measurement1/LConn2 -- Ground64/LConn1 -- Controlled Current Source/LConn1

== system ng_pv_dynamic_dbus_p_1_sm_ng/SM_NG/Single-Phase Dynamic Load55 ==
  PQ : Inport
  Controlled Current Source : powerlib/Electrical Sources/Controlled Current Source  Initialize=on  Source_Type=AC  Amplitude=0  Phase=0  Frequency=0  Measurements=None
  Ground62 : powerlib/Elements/Ground  LConnTagsString=a
  Voltage Measurement1 : powerlib/Measurements/Voltage Measurement  PhasorSimulation=off  OutputType=Complex  PSBequivalent=0
  model : Subsystem
  a : PMIOPort  Tag=PMCPort  Port=1  Side=Right
  wires:
  PQ/1 -> model/2(PQ)
  Voltage Measurement1/1 -> model/1(v)
  model/1(i) -> Controlled Current Source/1
  connections:
  Voltage Measurement1/LConn1 -- a/RConn1 -- Controlled Current Source/RConn1
  Voltage Measurement1/LConn2 -- Ground62/LConn1 -- Controlled Current Source/LConn1

== system ng_pv_dynamic_dbus_p_1_sm_ng/SM_NG/Single-Phase Dynamic Load56 ==
  PQ : Inport
  Controlled Current Source : powerlib/Electrical Sources/Controlled Current Source  Initialize=on  Source_Type=AC  Amplitude=0  Phase=0  Frequency=0  Measurements=None
  Ground50 : powerlib/Elements/Ground  LConnTagsString=a
  Voltage Measurement1 : powerlib/Measurements/Voltage Measurement  PhasorSimulation=off  OutputType=Complex  PSBequivalent=0
  model : Subsystem
  a : PMIOPort  Tag=PMCPort  Port=1  Side=Right
  wires:
  PQ/1 -> model/2(PQ)
  Voltage Measurement1/1 -> model/1(v)
  model/1(i) -> Controlled Current Source/1
  connections:
  Voltage Measurement1/LConn1 -- a/RConn1 -- Controlled Current Source/RConn1
  Voltage Measurement1/LConn2 -- Ground50/LConn1 -- Controlled Current Source/LConn1

== system ng_pv_dynamic_dbus_p_1_sm_ng/SM_NG/Single-Phase Dynamic Load57 ==
  PQ : Inport
  Controlled Current Source : powerlib/Electrical Sources/Controlled Current Source  Initialize=on  Source_Type=AC  Amplitude=0  Phase=0  Frequency=0  Measurements=None
  Ground51 : powerlib/Elements/Ground  LConnTagsString=a
  Voltage Measurement1 : powerlib/Measurements/Voltage Measurement  PhasorSimulation=off  OutputType=Complex  PSBequivalent=0
  model : Subsystem
  a : PMIOPort  Tag=PMCPort  Port=1  Side=Right
  wires:
  PQ/1 -> model/2(PQ)
  Voltage Measurement1/1 -> model/1(v)
  model/1(i) -> Controlled Current Source/1
  connections:
  Voltage Measurement1/LConn1 -- a/RConn1 -- Controlled Current Source/RConn1
  Voltage Measurement1/LConn2 -- Ground51/LConn1 -- Controlled Current Source/LConn1

== system ng_pv_dynamic_dbus_p_1_sm_ng/SM_NG/Single-Phase Dynamic Load58 ==
  PQ : Inport
  Controlled Current Source : powerlib/Electrical Sources/Controlled Current Source  Initialize=on  Source_Type=AC  Amplitude=0  Phase=0  Frequency=0  Measurements=None
  Ground51 : powerlib/Elements/Ground  LConnTagsString=a
  Voltage Measurement1 : powerlib/Measurements/Voltage Measurement  PhasorSimulation=off  OutputType=Complex  PSBequivalent=0
  model : Subsystem
  a : PMIOPort  Tag=PMCPort  Port=1  Side=Right
  wires:
  PQ/1 -> model/2(PQ)
  Voltage Measurement1/1 -> model/1(v)
  model/1(i) -> Controlled Current Source/1
  connections:
  Voltage Measurement1/LConn1 -- a/RConn1 -- Controlled Current Source/RConn1
  Voltage Measurement1/LConn2 -- Ground51/LConn1 -- Controlled Current Source/LConn1

== system ng_pv_dynamic_dbus_p_1_sm_ng/SM_NG/Single-Phase Dynamic Load59 ==
  PQ : Inport
  Controlled Current Source : powerlib/Electrical Sources/Controlled Current Source  Initialize=on  Source_Type=AC  Amplitude=0  Phase=0  Frequency=0  Measurements=None
  Ground51 : powerlib/Elements/Ground  LConnTagsString=a
  Voltage Measurement1 : powerlib/Measurements/Voltage Measurement  PhasorSimulation=off  OutputType=Complex  PSBequivalent=0
  model : Subsystem
  a : PMIOPort  Tag=PMCPort  Port=1  Side=Right
  wires:
  PQ/1 -> model/2(PQ)
  Voltage Measurement1/1 -> model/1(v)
  model/1(i) -> Controlled Current Source/1
  connections:
  Voltage Measurement1/LConn1 -- a/RConn1 -- Controlled Current Source/RConn1
  Voltage Measurement1/LConn2 -- Controlled Current Source/LConn1 -- Ground51/LConn1

== system ng_pv_dynamic_dbus_p_1_sm_ng/SM_NG/Single-Phase Dynamic Load60 ==
  PQ : Inport
  Controlled Current Source : powerlib/Electrical Sources/Controlled Current Source  Initialize=on  Source_Type=AC  Amplitude=0  Phase=0  Frequency=0  Measurements=None
  Ground52 : powerlib/Elements/Ground  LConnTagsString=a
  Voltage Measurement1 : powerlib/Measurements/Voltage Measurement  PhasorSimulation=off  OutputType=Complex  PSBequivalent=0
  model : Subsystem
  a : PMIOPort  Tag=PMCPort  Port=1  Side=Right
  wires:
  PQ/1 -> model/2(PQ)
  Voltage Measurement1/1 -> model/1(v)
  model/1(i) -> Controlled Current Source/1
  connections:
  Voltage Measurement1/LConn1 -- a/RConn1 -- Controlled Current Source/RConn1
  Voltage Measurement1/LConn2 -- Ground52/LConn1 -- Controlled Current Source/LConn1

== system ng_pv_dynamic_dbus_p_1_sm_ng/SM_NG/Subsystem ==
  Single-Phase Voltage Regulator1 : Subsystem  mask(Single-Phase Voltage Regulator){pNom=3330e3, fNom=60, vNom=13.8e3/sqrt(3), rFdrCurrent=3330e3/(13.8e3*sqrt(3)), iTapNo=0, vRef=122.4/120, bandwidth=1.25, totalDelay=30, rComp=6, xComp=6}
      mask prompts: pNom "Nominal power (VA)"; fNom "Nominal frequency (Hz)"; vNom "Nominal voltage (Vrms)"; rFdrCurrent "Rated feeder current (A)"; iTapNo "Initial tap number (-17 < x < 17)"; vRef "Reference voltage (P.U.)"; bandwidth "Bandwidth (P.U.)"; totalDelay "Time delay (s) + mechanical delay (s)"; rComp "R (V)"; xComp "X (V)"
      mask help:
      | The single-phase VR is designed for MV and primary LV systems. It consists of a 16-tap autotransformer and a step voltage regulating relay.
      |
      | The VR contains a reversing switch enabling a +/- 10% regulating range, in 16 steps up and 16 steps down.
      |
      | The VR performs a tap change if:
      |     abs(V-Vref) > Bandwidth/2  during a time  t > total delay.
      |
      | Note that R and X, specified on the "Compensator Settings" tab, are needed to dial on the control box of the regulator and are in units of volts.
      |
      | More info on VR modeling:
      |     W. H. Kersting, ribution Feeder Voltage Regulation Control,6, March/April 2010.
      mask init:
      | ptRatio = vNom / 120;  % Compensator and logic circuits are rated for 120V. 
      | ctRatio = rFdrCurrent / 0.2;  % The rated secondary current is 0.2A.
      | 
      | % Since the rated secondary current of the CT is 0.2A, the impedance of the
      | % analog compensator is obtained from the following equations to result in
      | % the voltage drop specified by Zcomp.
      | r = rComp / 0.2;   
      | x = xComp / 0.2;
      mask Display: image(imread('VR.jpg'))
  Single-Phase Voltage Regulator2 : Subsystem  mask(Single-Phase Voltage Regulator){pNom=3330e3, fNom=60, vNom=13.8e3/sqrt(3), rFdrCurrent=3330e3/(13.8e3*sqrt(3)), iTapNo=-2, vRef=122.4/120, bandwidth=1.25, totalDelay=30, rComp=6, xComp=6}
      mask prompts: pNom "Nominal power (VA)"; fNom "Nominal frequency (Hz)"; vNom "Nominal voltage (Vrms)"; rFdrCurrent "Rated feeder current (A)"; iTapNo "Initial tap number (-17 < x < 17)"; vRef "Reference voltage (P.U.)"; bandwidth "Bandwidth (P.U.)"; totalDelay "Time delay (s) + mechanical delay (s)"; rComp "R (V)"; xComp "X (V)"
      mask help:
      | The single-phase VR is designed for MV and primary LV systems. It consists of a 16-tap autotransformer and a step voltage regulating relay.
      |
      | The VR contains a reversing switch enabling a +/- 10% regulating range, in 16 steps up and 16 steps down.
      |
      | The VR performs a tap change if:
      |     abs(V-Vref) > Bandwidth/2  during a time  t > total delay.
      |
      | Note that R and X, specified on the "Compensator Settings" tab, are needed to dial on the control box of the regulator and are in units of volts.
      |
      | More info on VR modeling:
      |     W. H. Kersting, ribution Feeder Voltage Regulation Control,6, March/April 2010.
      mask init: same as ng_pv_dynamic_dbus_p_1_sm_ng/SM_NG/Subsystem/Single-Phase Voltage Regulator1
      mask Display: image(imread('VR.jpg'))
  Single-Phase Voltage Regulator3 : Subsystem  mask(Single-Phase Voltage Regulator){pNom=3330e3, fNom=60, vNom=13.8e3/sqrt(3), rFdrCurrent=3330e3/(13.8e3*sqrt(3)), iTapNo=0, vRef=122.4/120, bandwidth=1.25, totalDelay=30, rComp=6, xComp=6}
      mask prompts: pNom "Nominal power (VA)"; fNom "Nominal frequency (Hz)"; vNom "Nominal voltage (Vrms)"; rFdrCurrent "Rated feeder current (A)"; iTapNo "Initial tap number (-17 < x < 17)"; vRef "Reference voltage (P.U.)"; bandwidth "Bandwidth (P.U.)"; totalDelay "Time delay (s) + mechanical delay (s)"; rComp "R (V)"; xComp "X (V)"
      mask help:
      | The single-phase VR is designed for MV and primary LV systems. It consists of a 16-tap autotransformer and a step voltage regulating relay.
      |
      | The VR contains a reversing switch enabling a +/- 10% regulating range, in 16 steps up and 16 steps down.
      |
      | The VR performs a tap change if:
      |     abs(V-Vref) > Bandwidth/2  during a time  t > total delay.
      |
      | Note that R and X, specified on the "Compensator Settings" tab, are needed to dial on the control box of the regulator and are in units of volts.
      |
      | More info on VR modeling:
      |     W. H. Kersting, ribution Feeder Voltage Regulation Control,6, March/April 2010.
      mask init: same as ng_pv_dynamic_dbus_p_1_sm_ng/SM_NG/Subsystem/Single-Phase Voltage Regulator1
      mask Display: image(imread('VR.jpg'))
  Conn1 : PMIOPort  Port=1  Side=Left
  Conn2 : PMIOPort  Port=2  Side=Right
  Conn3 : PMIOPort  Port=3  Side=Left
  Conn4 : PMIOPort  Port=4  Side=Right
  Conn5 : PMIOPort  Port=5  Side=Left
  Conn6 : PMIOPort  Port=6  Side=Right
  Out1 : Outport
  Out2 : Outport  Port=2
  Out3 : Outport  Port=3
  wires:
  Single-Phase Voltage Regulator3/1(tapNo) -> Out1/1
  Single-Phase Voltage Regulator1/1(tapNo) -> Out3/1
  Single-Phase Voltage Regulator2/1(tapNo) -> Out2/1
  connections:
  Conn4/RConn1 -- Single-Phase Voltage Regulator2/RConn1
  Conn6/RConn1 -- Single-Phase Voltage Regulator1/RConn1
  Conn2/RConn1 -- Single-Phase Voltage Regulator3/RConn1
  Single-Phase Voltage Regulator1/LConn1 -- Conn5/RConn1
  Single-Phase Voltage Regulator2/LConn1 -- Conn3/RConn1
  Single-Phase Voltage Regulator3/LConn1 -- Conn1/RConn1
